simulink model "lista3_item_e"  (R2014b)
settings: Solver=ode45  StartTime=0.0  StopTime=Tsim_e  RelTol=1e-3
values from neighbouring files (symbols this model uses):
  T = 1    [sistema_lista3.m]
libraries: cstblocks x3
settings Model: Creator=Danilo  LastModifiedBy=Danilo

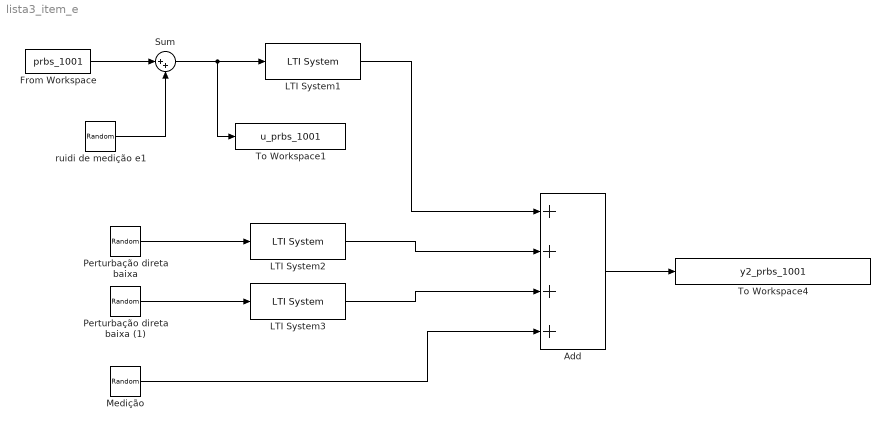
== system lista3_item_e ==
  Add : Sum  Inputs=++++
  From Workspace : FromWorkspace  VariableName=prbs_1001  SampleTime=T
  LTI System1 : cstblocks/LTI System  sys=H  IC=[]
  LTI System2 : cstblocks/LTI System  sys=G_pert_1  IC=[]
  LTI System3 : cstblocks/LTI System  sys=G_pert_2  IC=[]
  Medição : RandomNumber  Variance=exp(-6)  Seed=24  SampleTime=0.1
  Perturbação direta baixa : RandomNumber  Variance=0.001  SampleTime=0.1
  Perturbação direta baixa (1) : RandomNumber  Variance=0.001  Seed=12  SampleTime=0.1
  Sum : Sum  Inputs=|++
  To Workspace1 : ToWorkspace  VariableName=u_prbs_1001  SampleTime=T
  To Workspace4 : ToWorkspace  VariableName=y2_prbs_1001  SampleTime=T
  "ruidi de medição e1 " : RandomNumber  Variance=exp(-6)  SampleTime=0.1
  wires:
  LTI System1/1 -> Add/1
  Add/1 -> To Workspace4/1
  Perturbação direta baixa/1 -> LTI System2/1
  Perturbação direta baixa (1)/1 -> LTI System3/1
  LTI System2/1 -> Add/2
  LTI System3/1 -> Add/3
  Medição/1 -> Add/4
  From Workspace/1 -> Sum/1
  Sum/1 -> To Workspace1/1, LTI System1/1
  "ruidi de medição e1 "/1 -> Sum/2
